simulink model "test_approx_modele6"  (R2024a)
settings: Solver=VariableStepAuto  StartTime=0.0  StopTime=110  RelTol=1e-3
values from neighbouring files (symbols this model uses):
  K = -(9.5-ampli_ent)    (= -8.5)    [etablissement_variables.m]
  K_voulu = 1    [etablissement_variables.m]
  omega_n = 5/t5    (= 0.0919117647059)    [etablissement_variables.m]
  omega_n_voulu = 5/t5_voulu    (= 50)    [etablissement_variables.m]
  z = 1    [etablissement_variables.m]
  z_voulu = 1    [etablissement_variables.m]
settings Model: Creator=TP-EEA  LastModifiedBy=TP-EEA

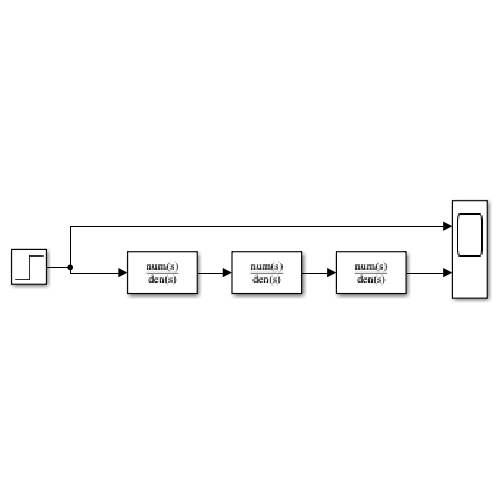
[thumbnail: Simulink's stored preview of the top-level diagram]
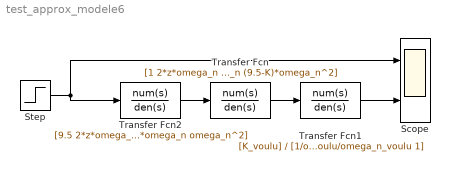
== system test_approx_modele6 ==
  Scope : Scope  NumInputPorts=2
  Step : Step  Time=0  SampleTime=0
  Transfer Fcn : TransferFcn  Numerator=[1 2*z*omega_n omega_n^2]  Denominator=[9.5 2*z*omega_n (9.5-K)*omega_n^2]
  Transfer Fcn1 : TransferFcn  Numerator=[K_voulu]  Denominator=[1/omega_n_voulu^2 2*z_voulu/omega_n_voulu 1]
  Transfer Fcn2 : TransferFcn  Numerator=[9.5 2*z*omega_n (9.5-K)*omega_n^2]  Denominator=[1 2*z*omega_n omega_n^2]
  wires:
  Step/1 -> Scope/1, Transfer Fcn2/1
  Transfer Fcn/1 -> Transfer Fcn1/1
  Transfer Fcn1/1 -> Scope/2
  Transfer Fcn2/1 -> Transfer Fcn/1
